simulink model "Problem_2"  (R2020a)
settings: Solver=VariableStepAuto  StartTime=0.0  StopTime=10.0  RelTol=1e-3
model workspace (MAT data in the model file):
  Fn = 20
  Ie = 1
  Iv = 5
  R = 1
  Tin = 100
  be = 1
  bv = 2
  mu_k = 1
  mu_s = 1.5
settings Model: Creator=Shubham Singh Rathor  LastModifiedBy=Shubham Singh Rathor

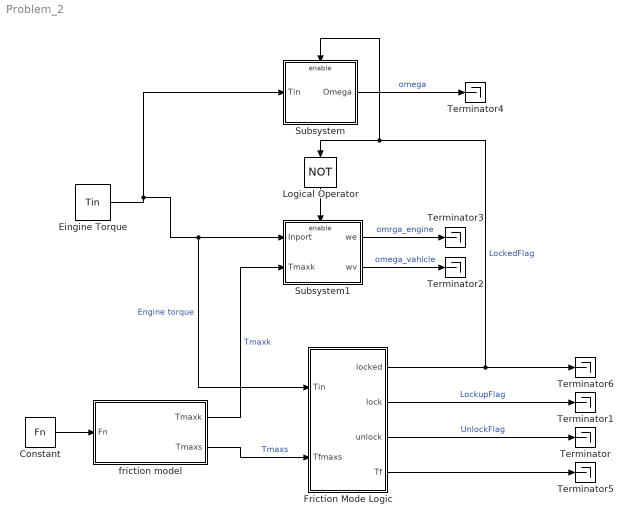
== system Problem_2 ==
  Constant : Constant  Value=Fn
  Eingine Torque : Constant  Value=Tin
  Friction Mode Logic : Subsystem
      mask Display: plot([-3 1 1 3 -1 -1],[-1 -1 1 1 1 -1],-4,-5,4,5)
  Logical Operator : Logic  Operator=NOT  IconShape=distinctive  AllPortsSameDT=off  OutDataTypeStr=boolean
  Subsystem : Subsystem
  Subsystem1 : Subsystem
  Terminator{,1..6} (7 alike) : Terminator
  friction model : Subsystem
  wires:
  Subsystem/1(Omega) -> Terminator4/1  "omega"
  Subsystem1/1(we) -> Terminator3/1  "omrga_engine"
  Subsystem1/2(wv) -> Terminator2/1  "omega_vahicle"
  Eingine Torque/1 -> Subsystem/1(Tin), Friction Mode Logic/1(Tin), Subsystem1/1(Inport)  "Engine torque"
  Logical Operator/1 -> Subsystem1/Enable
  Friction Mode Logic/1(locked) -> Terminator6/1, Logical Operator/1, Subsystem/Enable  "LockedFlag"
  friction model/2(Tmaxs) -> Friction Mode Logic/2(Tfmaxs)  "Tmaxs"
  friction model/1(Tmaxk) -> Subsystem1/2(Tmaxk)  "Tmaxk"
  Constant/1 -> friction model/1(Fn)
  Friction Mode Logic/2(lock) -> Terminator1/1  "LockupFlag"
  Friction Mode Logic/3(unlock) -> Terminator/1  "UnlockFlag"
  Friction Mode Logic/4(Tf) -> Terminator5/1

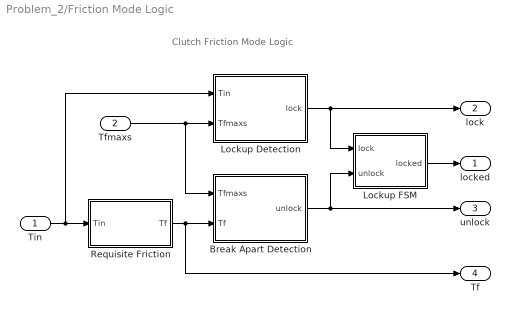
== system Problem_2/Friction Mode Logic ==
  note: Clutch Friction Mode Logic
  Tin : Inport
  Tfmaxs : Inport  Port=2
  Break Apart Detection : Subsystem
  Lockup Detection : Subsystem
  Lockup FSM : Subsystem
  Requisite Friction : Subsystem
  locked : Outport  InitialOutput=0  VectorParamsAs1DForOutWhenUnconnected=off
  lock : Outport  Port=2  InitialOutput=0  VectorParamsAs1DForOutWhenUnconnected=off
  unlock : Outport  Port=3  InitialOutput=0  VectorParamsAs1DForOutWhenUnconnected=off
  Tf : Outport  Port=4  InitialOutput=0  VectorParamsAs1DForOutWhenUnconnected=off
  wires:
  Tin/1 -> Lockup Detection/1(Tin), Requisite Friction/1(Tin)
  Tfmaxs/1 -> Lockup Detection/2(Tfmaxs), Break Apart Detection/1(Tfmaxs)
  Requisite Friction/1(Tf) -> Break Apart Detection/2(Tf), Tf/1
  Break Apart Detection/1(unlock) -> Lockup FSM/2(unlock), unlock/1
  Lockup Detection/1(lock) -> Lockup FSM/1(lock), lock/1
  Lockup FSM/1(locked) -> locked/1

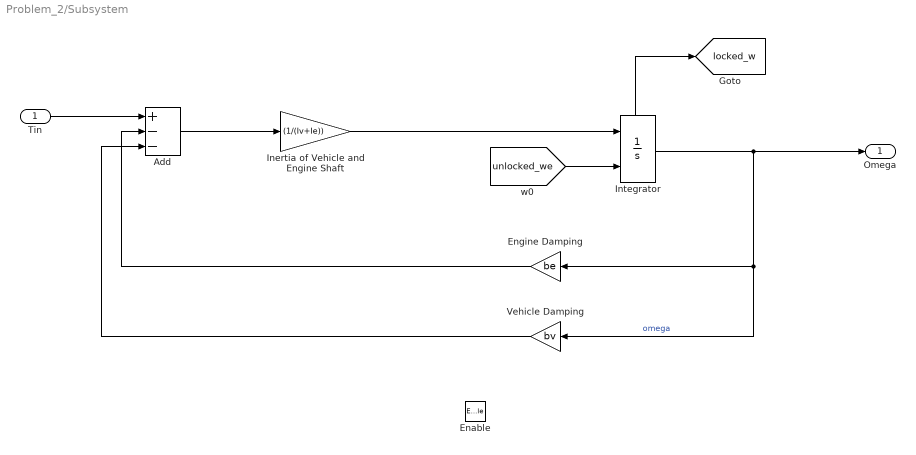
== system Problem_2/Subsystem ==
  Tin : Inport
  Enable : EnablePort
  Add : Sum  Inputs=+--
  Engine Damping : Gain  Gain=be
  Inertia of Vehicle and Engine Shaft : Gain  Gain=(1/(Iv+Ie))
  Integrator : Integrator  InitialConditionSource=external  ShowStatePort=on
  Vehicle Damping : Gain  Gain=bv
  Omega : Outport
  tag scope: locked_w=global
  wires:
  Integrator/1 -> Omega/1, Vehicle Damping/1, Engine Damping/1  "omega"
  Tin/1 -> Add/1
  [unlocked_we] -> Integrator/2
  Integrator/State -> [locked_w]
  Add/1 -> Inertia of Vehicle and Engine Shaft/1
  Inertia of Vehicle and Engine Shaft/1 -> Integrator/1
  Engine Damping/1 -> Add/2
  Vehicle Damping/1 -> Add/3

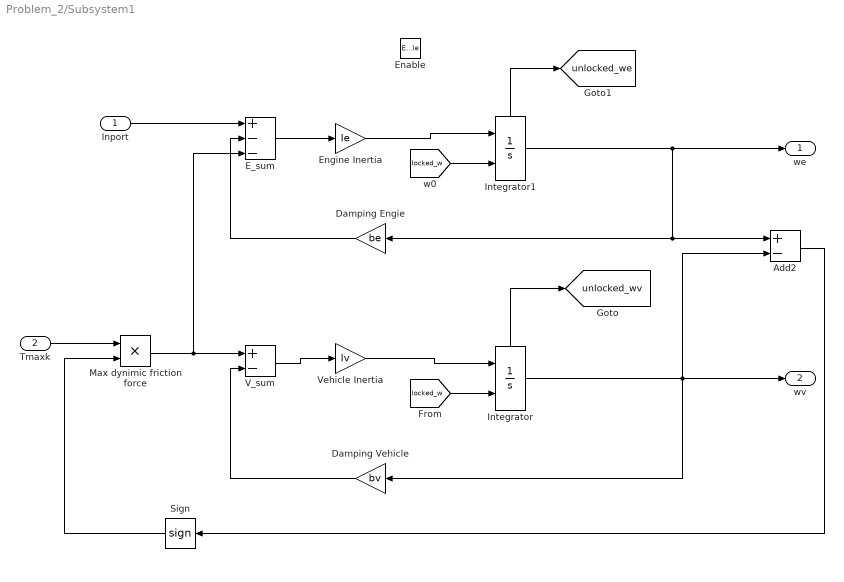
== system Problem_2/Subsystem1 ==
  Inport : Inport
  Tmaxk : Inport  Port=2
  Enable : EnablePort
  Add2 : Sum  Inputs=+-
  Damping Engie : Gain  Gain=be
  Damping Vehicle : Gain  Gain=bv
  E_sum : Sum  Inputs=+--
  Engine Inertia : Gain  Gain=Ie
  Integrator : Integrator  InitialConditionSource=external  ShowStatePort=on
  Integrator1 : Integrator  InitialConditionSource=external  ShowStatePort=on
  Max dynimic friction force : Product
  Sign : Signum
  V_sum : Sum  Inputs=+-
  Vehicle Inertia : Gain  Gain=Iv
  we : Outport
  wv : Outport  Port=2
  tag scope: unlocked_we=global, unlocked_wv=global
  wires:
  V_sum/1 -> Vehicle Inertia/1
  Integrator/1 -> wv/1, Damping Vehicle/1, Add2/2
  Damping Engie/1 -> E_sum/2
  Integrator1/1 -> we/1, Add2/1, Damping Engie/1
  Integrator/State -> [unlocked_wv]
  E_sum/1 -> Engine Inertia/1
  Engine Inertia/1 -> Integrator1/1
  Vehicle Inertia/1 -> Integrator/1
  Damping Vehicle/1 -> V_sum/2
  [locked_w] -> Integrator/2
  Max dynimic friction force/1 -> E_sum/3, V_sum/1
  [locked_w] -> Integrator1/2
  Integrator1/State -> [unlocked_we]
  Inport/1 -> E_sum/1
  Add2/1 -> Sign/1
  Tmaxk/1 -> Max dynimic friction force/1
  Sign/1 -> Max dynimic friction force/2

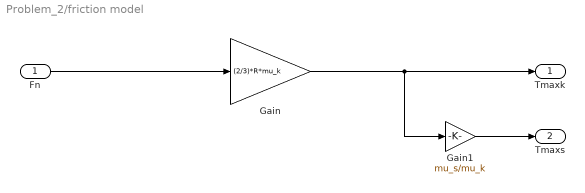
== system Problem_2/friction model ==
  Fn : Inport
  Gain : Gain  Gain=(2/3)*R*mu_k
  Gain1 : Gain  Gain=mu_s/mu_k
  Tmaxk : Outport
  Tmaxs : Outport  Port=2
  wires:
  Fn/1 -> Gain/1
  Gain/1 -> Tmaxk/1, Gain1/1
  Gain1/1 -> Tmaxs/1

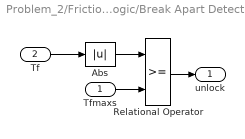
== system Problem_2/Friction Mode Logic/Break Apart Detection ==
  Tfmaxs : Inport
  Tf : Inport  Port=2
  Abs : Abs  SaturateOnIntegerOverflow=on
  Relational Operator : RelationalOperator  OutDataTypeStr=boolean  RndMeth=Nearest  InputSameDT=on
  unlock : Outport  InitialOutput=0  VectorParamsAs1DForOutWhenUnconnected=off
  wires:
  Tf/1 -> Abs/1
  Relational Operator/1 -> unlock/1
  Abs/1 -> Relational Operator/1
  Tfmaxs/1 -> Relational Operator/2

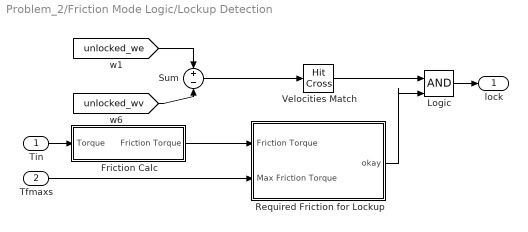
== system Problem_2/Friction Mode Logic/Lockup Detection ==
  Tin : Inport
  Tfmaxs : Inport  Port=2
  Friction Calc : Subsystem
  Logic : Logic  IconShape=distinctive  OutDataTypeStr=boolean
  Required Friction for Lockup : Subsystem
  Sum : Sum  Inputs=+-  InputSameDT=on  SaturateOnIntegerOverflow=on  OutDataTypeStr=Inherit: Same as first input
  Velocities Match : HitCross
  lock : Outport  InitialOutput=0  VectorParamsAs1DForOutWhenUnconnected=off
  wires:
  Friction Calc/1(Friction Torque) -> Required Friction for Lockup/1(Friction Torque)
  Tfmaxs/1 -> Required Friction for Lockup/2(Max Friction Torque)
  Velocities Match/1 -> Logic/1
  Logic/1 -> lock/1
  Required Friction for Lockup/1(okay) -> Logic/2
  [unlocked_we] -> Sum/1
  [unlocked_wv] -> Sum/2
  Sum/1 -> Velocities Match/1
  Tin/1 -> Friction Calc/1(Torque)

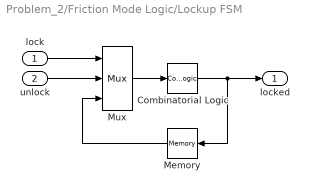
== system Problem_2/Friction Mode Logic/Lockup FSM ==
  lock : Inport
  unlock : Inport  Port=2
  Combinatorial Logic : CombinatorialLogic  TruthTable=[0;1;0;0;1;1;1;0]
  Memory : Memory
  Mux : Mux  Inputs=3
  locked : Outport  InitialOutput=0  VectorParamsAs1DForOutWhenUnconnected=off
  wires:
  Memory/1 -> Mux/3
  Combinatorial Logic/1 -> locked/1, Memory/1
  unlock/1 -> Mux/2
  lock/1 -> Mux/1
  Mux/1 -> Combinatorial Logic/1

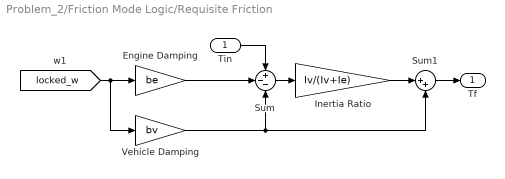
== system Problem_2/Friction Mode Logic/Requisite Friction ==
  Tin : Inport
  Engine Damping : Gain  Gain=be  SaturateOnIntegerOverflow=on  OutDataTypeStr=Inherit: Same as input  ParamDataTypeStr=Inherit: Same as input
  Inertia Ratio : Gain  Gain=Iv/(Iv+Ie)  SaturateOnIntegerOverflow=on  OutDataTypeStr=Inherit: Same as input  ParamDataTypeStr=Inherit: Same as input
  Sum : Sum  Inputs=+--  InputSameDT=on  SaturateOnIntegerOverflow=on  OutDataTypeStr=Inherit: Same as first input
  Sum1 : Sum  Inputs=|++  InputSameDT=on  SaturateOnIntegerOverflow=on  OutDataTypeStr=Inherit: Same as first input
  Vehicle Damping : Gain  Gain=bv  SaturateOnIntegerOverflow=on  OutDataTypeStr=Inherit: Same as input  ParamDataTypeStr=Inherit: Same as input
  Tf : Outport  InitialOutput=0  VectorParamsAs1DForOutWhenUnconnected=off
  wires:
  [locked_w] -> Vehicle Damping/1, Engine Damping/1
  Engine Damping/1 -> Sum/2
  Vehicle Damping/1 -> Sum/3, Sum1/2
  Sum/1 -> Inertia Ratio/1
  Tin/1 -> Sum/1
  Inertia Ratio/1 -> Sum1/1
  Sum1/1 -> Tf/1

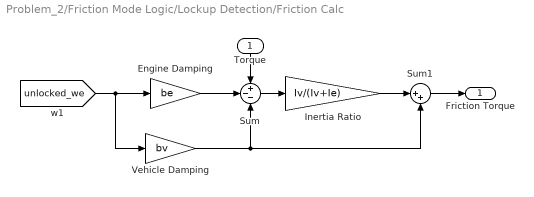
== system Problem_2/Friction Mode Logic/Lockup Detection/Friction Calc ==
  Torque : Inport
  Engine Damping : Gain  Gain=be  SaturateOnIntegerOverflow=on  OutDataTypeStr=Inherit: Same as input  ParamDataTypeStr=Inherit: Same as input
  Inertia Ratio : Gain  Gain=Iv/(Iv+Ie)  SaturateOnIntegerOverflow=on  OutDataTypeStr=Inherit: Same as input  ParamDataTypeStr=Inherit: Same as input
  Sum : Sum  Inputs=+--  InputSameDT=on  SaturateOnIntegerOverflow=on  OutDataTypeStr=Inherit: Same as first input
  Sum1 : Sum  Inputs=|++  InputSameDT=on  SaturateOnIntegerOverflow=on  OutDataTypeStr=Inherit: Same as first input
  Vehicle Damping : Gain  Gain=bv  SaturateOnIntegerOverflow=on  OutDataTypeStr=Inherit: Same as input  ParamDataTypeStr=Inherit: Same as input
  Friction Torque : Outport  InitialOutput=0  VectorParamsAs1DForOutWhenUnconnected=off
  wires:
  [unlocked_we] -> Engine Damping/1, Vehicle Damping/1
  Vehicle Damping/1 -> Sum1/2, Sum/3
  Engine Damping/1 -> Sum/2
  Sum/1 -> Inertia Ratio/1
  Torque/1 -> Sum/1
  Inertia Ratio/1 -> Sum1/1
  Sum1/1 -> Friction Torque/1

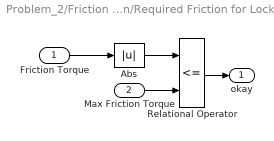
== system Problem_2/Friction Mode Logic/Lockup Detection/Required Friction for Lockup ==
  Friction Torque : Inport
  Max Friction Torque : Inport  Port=2
  Abs : Abs  SaturateOnIntegerOverflow=on
  Relational Operator : RelationalOperator  Operator=<=  OutDataTypeStr=boolean  RndMeth=Nearest  InputSameDT=on
  okay : Outport  InitialOutput=0  VectorParamsAs1DForOutWhenUnconnected=off
  wires:
  Friction Torque/1 -> Abs/1
  Relational Operator/1 -> okay/1
  Abs/1 -> Relational Operator/1
  Max Friction Torque/1 -> Relational Operator/2
